simulink model "prob2bias"  (R2019a)
settings: Solver=VariableStepAuto  StartTime=0.0  StopTime=10.0  RelTol=1e-3
values from neighbouring files (symbols this model uses):
  altBias = altBiases(1)    [prob2main.m]
  bias = 1E-3 * g    [prob2main.m]
  C1 = 2 / tau    [prob2main.m]
  C2 = 1/tau/tau + 2 * schuler^2    [prob2main.m]
  schuler = sqrt(g/R)    [prob2main.m]
settings Model: Creator=hyunwoong  LastModifiedBy=hyunwoong

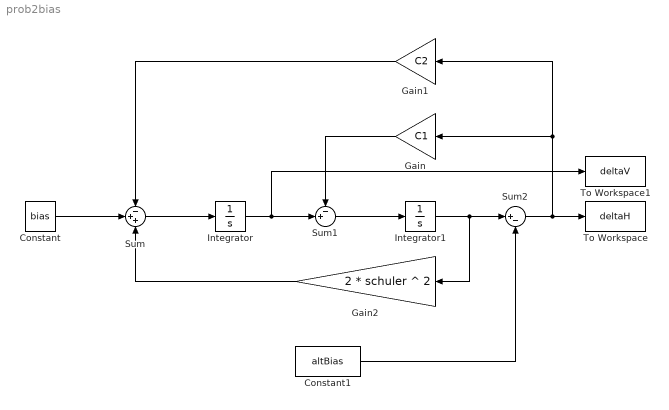
== system prob2bias ==
  Constant : Constant  Value=bias
  Constant1 : Constant  Value=altBias
  Gain : Gain  Gain=C1
  Gain1 : Gain  Gain=C2
  Gain2 : Gain  Gain=2 * schuler ^ 2
  Integrator : Integrator
  Integrator1 : Integrator
  Sum : Sum  Inputs=-++
  Sum1 : Sum  Inputs=-+|
  Sum2 : Sum  Inputs=|+-
  To Workspace : ToWorkspace  VariableName=deltaH  SaveFormat=Timeseries  SampleTime=-1
  To Workspace1 : ToWorkspace  VariableName=deltaV  SaveFormat=Timeseries  SampleTime=-1
  wires:
  Sum/1 -> Integrator/1
  Integrator/1 -> To Workspace1/1, Sum1/2
  Sum1/1 -> Integrator1/1
  Integrator1/1 -> Sum2/1, Gain2/1
  Sum2/1 -> To Workspace/1, Gain1/1, Gain/1
  Gain/1 -> Sum1/1
  Gain1/1 -> Sum/1
  Gain2/1 -> Sum/3
  Constant1/1 -> Sum2/2
  Constant/1 -> Sum/2
